simulink model "testemplanner_cs"  (R2023a)
settings: Solver=ode5  StartTime=0.0  StopTime=60  FixedStep=1/1000  RelTol=1e-3
PreLoadFcn:
  | mbxruntime.callbacks.PreLoadFcn(bdroot);
PostLoadFcn:
  | mbxruntime.callbacks.PostLoadFcn(bdroot);
InitFcn:
  | mbxruntime.callbacks.InitFcn(bdroot);
StartFcn:
  | mbxruntime.callbacks.StartFcn(bdroot);
StopFcn:
  | mbxruntime.callbacks.StopFcn(bdroot);
model workspace (MAT data in the model file):
  mbox_table : object (value not decoded)
  model_closed = 0
  sim_status = 0
undefined symbols (not defined in the file): aubr, c_factor, cf, cr, DiscIntNeverNeededParam, global_path_x, global_path_y, KD_PID_distance, KD_PID_speed, KI_PID_distance, KI_PID_speed, KP_PID_distance, KP_PID_speed, la, lb, LQR_K1, LQR_K2, LQR_K3, LQR_K4, m, rack_displacement, right_wheel_ground, tablebr, vubr, vx_break_point
libraries: PreScanSimulinkLibrary x14, Solver_SF x1
(part 4 of 8)

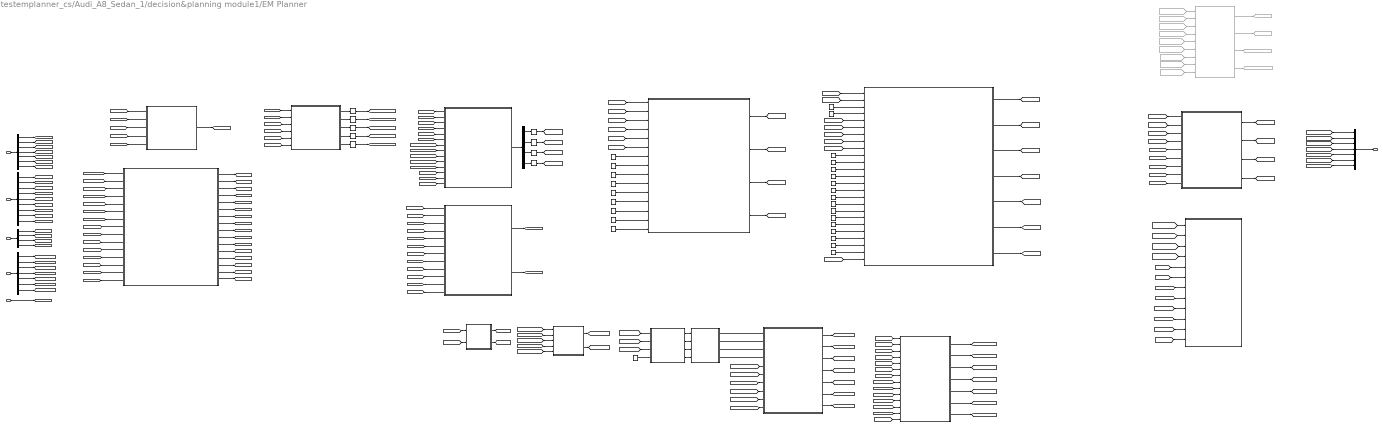
== system testemplanner_cs/Audi_A8_Sedan_1/decision&planning module1/EM Planner ==
  referenceline_info : Inport
  location_info : Inport  Port=2
  perception_info : Inport  Port=3
  pre_planning_info : Inport  Port=4
  current time : Inport  Port=5
  Bus Creator : BusCreator  Inputs=7
  Bus Selector : BusSelector  OutputSignals=referenceline_x,referenceline_y,referenceline_heading,referenceline_kappa,origin_match_point_index,origin_proj_x,origin_proj_y
  Bus Selector1 : BusSelector  OutputSignals=host_x,host_y,host_heading_xy,host_vx,host_vy,host_yawrate,host_speed,host_ax,host_ay
  Bus Selector2 : BusSelector  OutputSignals=obs_x_set_gcs,obs_y_set_gcs,obs_velocity_set_gcs,obs_heading_set_gcs
  Bus Selector3 : BusSelector  OutputSignals=trajectory_x_gcs,trajectory_y_gcs,trajectory_heading_gcs,trajectory_kappa_gcs,trajectory_speed_gcs,trajectory_accel_gcs,trajectory_time_gcs
  Bus Selector4 : BusSelector  OutputSignals=s_set,l_set,dl_set,ddl_set
  Cartesian2Frenet-panning start point : Subsystem
  Constant : Constant  Value=11
  Constant1 : Constant  Value=4
  Constant10 : Constant  Value=5
  Constant11 : Constant  Value=2
  Constant12 : Constant  Value=2
  Constant13 : Constant  Value=25000
  Constant14 : Constant  Value=50
  Constant15 : Constant  Value=20
  Constant16 : Constant  Value=25
  Constant{2,17..19} (4 alike) : Constant  Value=15
  Constant20 : Constant  Value=3
  Constant21 : Constant  Value=3
  Constant22 : Constant  Value=1.63
  Constant23 : Constant  Value=0.1
  Constant24 : Constant  Value=-0.1
  Constant25 : Constant  Value=0.02
  Constant26 : Constant  Value=-0.02
  Constant3 : Constant
  Constant4 : Constant  Value=2000
  Constant5 : Constant  Value=2
  Constant6 : Constant  Value=3
  Constant7 : Constant  Value=10
  Constant8 : Constant  Value=1e6
  Constant9 : Constant  Value=8
  Dynamic Programming&Increase DP Node : Subsystem
  Frenet2Cartesian : MATLAB Function  TreatAsAtomicUnit=on
  Frenet2Cartesian task : MATLAB Function  Commented=on  TreatAsAtomicUnit=on
  From144 : From  Commented=on  GotoTag=qp_path_s
  From151 : From  Commented=on  GotoTag=qp_path_l
  From152 : From  Commented=on  GotoTag=qp_path_dl
  From153 : From  Commented=on  GotoTag=qp_path_ddl
  From154 : From  Commented=on  GotoTag=referenceline_x
  From155 : From  Commented=on  GotoTag=referenceline_y
  From156 : From  Commented=on  GotoTag=referenceline_heading
  From157 : From  Commented=on  GotoTag=referenceline_kappa
  From158 : From  Commented=on  GotoTag=index2s
  Generate Convex Space&Quadratic Programming : Subsystem
  Goto101 : Goto  Commented=on  GotoTag=trajectory_x_init
  Goto102 : Goto  Commented=on  GotoTag=trajectory_y_init
  Goto103 : Goto  Commented=on  GotoTag=trajectory_heading_init
  Goto104 : Goto  Commented=on  GotoTag=trajectory_kappa_init
  Obs : Subsystem
  Selector{1..9} (9 alike) : Selector  InputPortWidth=128  IndexOptions=Index vector (dialog)  Indices=1  OutputSizes=1
  cacul planning start gcs : MATLAB Function  TreatAsAtomicUnit=on
  calc path length and map between point and s : MATLAB Function  TreatAsAtomicUnit=on
  calc speed planning start condition : MATLAB Function  TreatAsAtomicUnit=on
  generate index2s : MATLAB Function  TreatAsAtomicUnit=on
  increase st point count : MATLAB Function  TreatAsAtomicUnit=on
  match&proj point search2 : MATLAB Function  TreatAsAtomicUnit=on
  path and speed merge : MATLAB Function  TreatAsAtomicUnit=on
  plot1 : MATLAB Function  TreatAsAtomicUnit=on
  simple speed qp planning : MATLAB Function  TreatAsAtomicUnit=on
  stitch trajectory : MATLAB Function  TreatAsAtomicUnit=on
  EM Planner result : Outport
  wires:
  referenceline_info/1 -> Bus Selector/1
  Bus Selector/1 -> [referenceline_x]  "<referenceline_x>"
  Bus Selector/2 -> [referenceline_y]  "<referenceline_y>"
  Bus Selector/3 -> [referenceline_heading]  "<referenceline_heading>"
  Bus Selector/4 -> [referenceline_kappa]  "<referenceline_kappa>"
  location_info/1 -> Bus Selector1/1
  Bus Selector1/1 -> [host_x]  "<host_x>"
  Bus Selector1/2 -> [host_y]  "<host_y>"
  Bus Selector1/3 -> [host_heading_xy]  "<host_heading_xy>"
  Bus Selector1/4 -> [host_vx_vcs]  "<host_vx>"
  Bus Selector1/5 -> [host_vy_vcs]  "<host_vy>"
  Bus Selector1/6 -> [host_yawrate]  "<host_yawrate>"
  Bus Selector1/7 -> [host_speed]  "<host_speed>"
  Bus Selector1/8 -> [host_ax_vcs]  "<host_ax>"
  Bus Selector1/9 -> [host_ay_vcs]  "<host_ay>"
  perception_info/1 -> Bus Selector2/1
  Bus Selector2/1 -> [obs_x_set_gcs]  "<obs_x_set_gcs>"
  Bus Selector2/2 -> [obs_y_set_gcs]  "<obs_y_set_gcs>"
  Bus Selector2/3 -> [obs_velocity_set_gcs]  "<obs_velocity_set_gcs>"
  Bus Selector2/4 -> [obs_heading_set_gcs]  "<obs_heading_set_gcs>"
  pre_planning_info/1 -> Bus Selector3/1
  Bus Selector3/1 -> [pre_trajectory_x_gcs]  "<trajectory_x_gcs>"
  Bus Selector3/2 -> [pre_trajectory_y_gcs]  "<trajectory_y_gcs>"
  Bus Selector3/3 -> [pre_trajectory_heading_gcs]  "<trajectory_heading_gcs>"
  Bus Selector3/4 -> [pre_trajectory_kappa_gcs]  "<trajectory_kappa_gcs>"
  Bus Selector3/5 -> [pre_trajectory_speed_gcs]  "<trajectory_speed_gcs>"
  Bus Selector3/6 -> [pre_trajectory_accel_gcs]  "<trajectory_accel_gcs>"
  current time/1 -> [current_time]
  [pre_trajectory_x_gcs] -> cacul planning start gcs/1(pre_trajectory_x)
  [pre_trajectory_y_gcs] -> cacul planning start gcs/2(pre_trajectory_y)
  [pre_trajectory_heading_gcs] -> cacul planning start gcs/3(pre_trajectory_heading)
  [pre_trajectory_kappa_gcs] -> cacul planning start gcs/4(pre_trajectory_kappa)
  [pre_trajectory_speed_gcs] -> cacul planning start gcs/5(pre_trajectory_speed)
  [pre_trajectory_accel_gcs] -> cacul planning start gcs/6(pre_trajectory_accel)
  [pre_trajectory_time] -> cacul planning start gcs/7(pre_trajectory_time)
  [current_time] -> cacul planning start gcs/8(current_time)
  [host_x] -> cacul planning start gcs/9(host_x)
  [host_y] -> cacul planning start gcs/10(host_y)
  [host_heading_xy] -> cacul planning start gcs/11(host_heading_xy)
  [host_vx_vcs] -> cacul planning start gcs/12(host_vx)
  [host_vy_vcs] -> cacul planning start gcs/13(host_vy)
  [host_ax_vcs] -> cacul planning start gcs/14(host_ax)
  [host_ay_vcs] -> cacul planning start gcs/15(host_ay)
  cacul planning start gcs/1(planning_start_x) -> [planning_start_x]
  cacul planning start gcs/2(planning_start_y) -> [planning_start_y]
  cacul planning start gcs/3(planning_start_heading) -> [planning_start_heading]
  cacul planning start gcs/4(planning_start_kappa) -> [planning_start_kappa]
  cacul planning start gcs/5(planning_start_vx) -> [planning_start_vx]
  cacul planning start gcs/6(planning_start_vy) -> [planning_start_vy]
  cacul planning start gcs/7(planning_start_ax) -> [planning_start_ax]
  cacul planning start gcs/8(planning_start_ay) -> [planning_start_ay]
  cacul planning start gcs/9(planning_start_time) -> [planning_start_time]
  cacul planning start gcs/10(stitch_x) -> [stitch_x]
  cacul planning start gcs/11(stitch_y) -> [stitch_y]
  cacul planning start gcs/12(stitch_heading) -> [stitch_heading]
  cacul planning start gcs/13(stitch_kappa) -> [stitch_kappa]
  cacul planning start gcs/14(stitch_speed) -> [stitch_speed]
  cacul planning start gcs/15(stitch_accel) -> [stitch_accel]
  cacul planning start gcs/16(stitch_time) -> [stitch_time]
  Bus Selector/5 -> [origin_match_point_index]  "<origin_match_point_index>"
  Bus Selector/6 -> [origin_proj_x]  "<origin_proj_x>"
  Bus Selector/7 -> [origin_proj_y]  "<origin_proj_y>"
  [origin_match_point_index] -> generate index2s/1(origin_match_point_index)
  [origin_proj_x] -> generate index2s/2(origin_proj_x)
  [origin_proj_y] -> generate index2s/3(origin_proj_y)
  [referenceline_x] -> generate index2s/4(path_x)
  [referenceline_y] -> generate index2s/5(path_y)
  generate index2s/1(index2s) -> [index2s]
  match&proj point search2/3(proj_y_set) -> Selector3/1
  match&proj point search2/1(match_point_index_set) -> Selector1/1
  match&proj point search2/2(proj_x_set) -> Selector2/1
  match&proj point search2/4(proj_heading_set) -> Selector4/1
  match&proj point search2/5(proj_kappa_set) -> Selector5/1
  [planning_start_x] -> match&proj point search2/1(x_set)
  [planning_start_y] -> match&proj point search2/2(y_set)
  [referenceline_x] -> match&proj point search2/3(frenet_x_set)
  [referenceline_y] -> match&proj point search2/4(frenet_y_set)
  [referenceline_heading] -> match&proj point search2/5(frenet_heading_set)
  [referenceline_kappa] -> match&proj point search2/6(frenet_kapppa_set)
  Selector1/1 -> [planning_start_match_point_index]
  Selector2/1 -> [planning_start_proj_x]
  Selector3/1 -> [planning_start_proj_y]
  Selector4/1 -> [planning_start_proj_heading]
  Selector5/1 -> [planning_start_proj_kappa]
  Cartesian2Frenet-panning start point/1(Caetesian2Frenetout) -> Bus Selector4/1
  Bus Selector4/1 -> Selector6/1  "<s_set>"
  Bus Selector4/2 -> Selector7/1  "<l_set>"
  Bus Selector4/3 -> Selector8/1  "<dl_set>"
  Bus Selector4/4 -> Selector9/1  "<ddl_set>"
  [planning_start_x] -> Cartesian2Frenet-panning start point/1(x_set)
  [planning_start_y] -> Cartesian2Frenet-panning start point/2(y_set)
  [planning_start_vx] -> Cartesian2Frenet-panning start point/3(vx_set)
  [planning_start_vy] -> Cartesian2Frenet-panning start point/4(vy_set)
  [planning_start_ax] -> Cartesian2Frenet-panning start point/5(ax_set)
  [planning_start_ay] -> Cartesian2Frenet-panning start point/6(ay_set)
  [planning_start_proj_x] -> Cartesian2Frenet-panning start point/7(proj_x_set)
  [planning_start_proj_y] -> Cartesian2Frenet-panning start point/8(proj_y_set)
  [planning_start_proj_heading] -> Cartesian2Frenet-panning start point/9(proj_heading_set)
  [planning_start_proj_kappa] -> Cartesian2Frenet-panning start point/10(proj_kappa_set)
  [planning_start_match_point_index] -> Cartesian2Frenet-panning start point/11(match_point_index_set)
  [referenceline_x] -> Cartesian2Frenet-panning start point/12(frenet_x_set)
  [referenceline_y] -> Cartesian2Frenet-panning start point/13(frenet_y_set)
  [index2s] -> Cartesian2Frenet-panning start point/14(index2s)
  Selector6/1 -> [planning_start_s]
  Selector7/1 -> [planning_start_l]
  Selector8/1 -> [planning_start_dl]
  Selector9/1 -> [planning_start_ddl]
  [host_x] -> Obs/1(host_x)
  [host_y] -> Obs/2(host_y)
  [obs_x_set_gcs] -> Obs/3(obs_x_set_gcs)
  [obs_y_set_gcs] -> Obs/4(obs_y_set_gcs)
  [obs_velocity_set_gcs] -> Obs/5(obs_velocity_set_gcs)
  [obs_heading_set_gcs] -> Obs/6(obs_heading_set_gcs)
  [host_heading_xy] -> Obs/7(host_heading_xy)
  [index2s] -> Obs/12(index2s)
  [referenceline_x] -> Obs/8(referenceline_x)
  [referenceline_y] -> Obs/9(referenceline_y)
  [referenceline_heading] -> Obs/10(referenceline_heading)
  [referenceline_kappa] -> Obs/11(referenceline_kappa)
  Obs/1(static_obs_s_set) -> [static_obs_s_set]
  Obs/2(static_obs_l_set) -> [static_obs_l_set]
  [qp_path_s] -> Frenet2Cartesian/1(s_set)
  [qp_path_l] -> Frenet2Cartesian/2(l_set)
  [qp_path_dl] -> Frenet2Cartesian/3(dl_set)
  [qp_path_ddl] -> Frenet2Cartesian/4(ddl_set)
  [referenceline_x] -> Frenet2Cartesian/5(frenet_x)
  [referenceline_y] -> Frenet2Cartesian/6(frenet_y)
  [referenceline_heading] -> Frenet2Cartesian/7(frenet_heading)
  [index2s] -> Frenet2Cartesian/9(index2s)
  [referenceline_kappa] -> Frenet2Cartesian/8(frenet_kappa)
  Frenet2Cartesian/1(x_point_set) -> [trajectory_x_init]
  Frenet2Cartesian/2(y_point_set) -> [trajectory_y_init]
  Frenet2Cartesian/3(heading_point_set) -> [trajectory_heading_init]
  Frenet2Cartesian/4(kappa_point_set) -> [trajectory_kappa_init]
  stitch trajectory/6(trajectory_accel_final) -> [trajectory_accel_final]
  stitch trajectory/7(trajectory_time_final) -> [trajectory_time_final]
  [trajectory_heading] -> stitch trajectory/3(trajectory_heading)
  [planning_start_time] -> path and speed merge/5(current_time)
  increase st point count/2(s_dot) -> path and speed merge/2(s_dot)
  [plan_start_s_dot] -> simple speed qp planning/1(plan_start_s_dot)
  [trajectory_x_final] -> Bus Creator/1  "trajectory_x_gcs"
  [stitch_kappa] -> stitch trajectory/11(stitch_kappa)
  [trajectory_y_final] -> Bus Creator/2  "trajectory_y_gcs"
  simple speed qp planning/4(relative_time_init) -> increase st point count/4(relative_time_init)
  path and speed merge/5(trajectory_speed) -> [trajectory_speed]
  simple speed qp planning/3(s_dot2_init) -> increase st point count/3(s_dot2_init)
  increase st point count/4(relative_time) -> path and speed merge/4(relative_time)
  [plan_start_s_dot2] -> simple speed qp planning/2(plan_start_s_dot2)
  simple speed qp planning/1(s_init) -> increase st point count/1(s_init)
  [trajectory_heading_init] -> path and speed merge/9(trajectory_heading_init)
  path and speed merge/7(trajectory_time) -> [trajectory_time]
  [trajectory_x] -> stitch trajectory/1(trajectory_x)
  path and speed merge/6(trajectory_accel) -> [trajectory_accel]
  [stitch_speed] -> stitch trajectory/12(stitch_speed)
  [trajectory_y] -> stitch trajectory/2(trajectory_y)
  [stitch_accel] -> stitch trajectory/13(stitch_accel)
  stitch trajectory/3(trajectory_heading_final) -> [trajectory_heading_final]
  [trajectory_x_init] -> path and speed merge/7(trajectory_x_init)
  [path_s] -> path and speed merge/6(path_s)
  [path_s_end] -> simple speed qp planning/3(s_end)
  calc speed planning start condition/2(plan_start_s_dot2) -> [plan_start_s_dot2]
  stitch trajectory/5(trajectory_speed_final) -> [trajectory_speed_final]
  Constant9/1 -> simple speed qp planning/4(recommend_T)
  [trajectory_time] -> stitch trajectory/7(trajectory_time)
  [stitch_time] -> stitch trajectory/14(stitch_time)
  [planning_start_ay] -> calc speed planning start condition/4(plan_start_ay)
  [trajectory_accel] -> stitch trajectory/6(trajectory_accel)
  [stitch_heading] -> stitch trajectory/10(stitch_heading)
  [trajectory_kappa] -> stitch trajectory/4(trajectory_kappa)
  [trajectory_heading_final] -> Bus Creator/3  "trajectory_heading_gcs"
  [trajectory_speed_final] -> Bus Creator/5  "trajectory_speed_gcs"
  increase st point count/3(s_dot2) -> path and speed merge/3(s_dot2)
  calc path length and map between point and s/2(path_s) -> [path_s]
  [trajectory_time_final] -> Bus Creator/7  "trajectory_time_gcs"
  stitch trajectory/4(trajectory_kappa_final) -> [trajectory_kappa_final]
  calc path length and map between point and s/1(path_s_end) -> [path_s_end]
  [planning_start_vy] -> calc speed planning start condition/2(plan_start_vy)
  increase st point count/1(s) -> path and speed merge/1(s)
  [planning_start_heading] -> calc speed planning start condition/5(plan_start_heading)
  [trajectory_accel_final] -> Bus Creator/6  "trajectory_accel_gcs"
  path and speed merge/4(trajectory_kappa) -> [trajectory_kappa]
  [stitch_y] -> stitch trajectory/9(stitch_y)
  path and speed merge/1(trajectory_x) -> [trajectory_x]
  stitch trajectory/1(trajectory_x_final) -> [trajectory_x_final]
  [trajectory_x_init] -> calc path length and map between point and s/1(trajectory_x)
  stitch trajectory/2(trajectory_y_final) -> [trajectory_y_final]
  calc speed planning start condition/1(plan_start_s_dot) -> [plan_start_s_dot]
  [trajectory_y_init] -> calc path length and map between point and s/2(trajectory_y)
  [trajectory_speed] -> stitch trajectory/5(trajectory_speed)
  [trajectory_kappa_init] -> path and speed merge/10(trajectory_kappa_init)
  [planning_start_vx] -> calc speed planning start condition/1(plan_start_vx)
  [trajectory_y_init] -> path and speed merge/8(trajectory_y_init)
  path and speed merge/2(trajectory_y) -> [trajectory_y]
  path and speed merge/3(trajectory_heading) -> [trajectory_heading]
  Bus Creator/1 -> EM Planner result/1
  [stitch_x] -> stitch trajectory/8(stitch_x)
  simple speed qp planning/2(s_dot_init) -> increase st point count/2(s_dot_init)
  [planning_start_ax] -> calc speed planning start condition/3(plan_start_ax)
  [trajectory_kappa_final] -> Bus Creator/4  "trajectory_kappa_gcs"
  Bus Selector3/7 -> [pre_trajectory_time]  "<trajectory_time_gcs>"
  From158/1 -> Frenet2Cartesian task/9(index2s)
  From156/1 -> Frenet2Cartesian task/7(frenet_path_heading)
  Frenet2Cartesian task/1(x_set) -> Goto101/1
  Frenet2Cartesian task/4(kappa_set) -> Goto104/1
  From157/1 -> Frenet2Cartesian task/8(frenet_path_kappa)
  Frenet2Cartesian task/2(y_set) -> Goto102/1
  From144/1 -> Frenet2Cartesian task/1(s_set)
  From154/1 -> Frenet2Cartesian task/5(frenet_path_x)
  From152/1 -> Frenet2Cartesian task/3(dl_set)
  From151/1 -> Frenet2Cartesian task/2(l_set)
  From155/1 -> Frenet2Cartesian task/6(frenet_path_y)
  From153/1 -> Frenet2Cartesian task/4(ddl_set)
  Frenet2Cartesian task/3(heading_set) -> Goto103/1
  [static_obs_s_set] -> plot1/7(obs_s_set)
  [planning_start_s] -> plot1/9(start_s)
  [l_min] -> plot1/5(l_min)
  [dp_path_l_final] -> plot1/2(dp_l)
  [planning_start_dl] -> plot1/11(start_dl)
  [dp_path_s_final] -> plot1/1(dp_s)
  [planning_start_l] -> plot1/10(start_l)
  [static_obs_l_set] -> plot1/8(obs_l_set)
  [qp_path_s] -> plot1/3(qp_s)
  [qp_path_l] -> plot1/4(qp_l)
  [l_max] -> plot1/6(l_max)
  [planning_start_s] -> Dynamic Programming&Increase DP Node/1(plan_start_s)
  [planning_start_l] -> Dynamic Programming&Increase DP Node/2(plan_start_l)
  [planning_start_dl] -> Dynamic Programming&Increase DP Node/3(plan_start_dl)
  [planning_start_ddl] -> Dynamic Programming&Increase DP Node/4(plan_start_ddl)
  [static_obs_s_set] -> Dynamic Programming&Increase DP Node/5(static_obs_s_set)
  [static_obs_l_set] -> Dynamic Programming&Increase DP Node/6(static_obs_l_set)
  Constant/1 -> Dynamic Programming&Increase DP Node/7(row)
  Constant1/1 -> Dynamic Programming&Increase DP Node/8(col)
  Constant2/1 -> Dynamic Programming&Increase DP Node/9(sample_s)
  Constant3/1 -> Dynamic Programming&Increase DP Node/10(sample_l)
  Constant4/1 -> Dynamic Programming&Increase DP Node/11(dp_dl_cost)
  Constant5/1 -> Dynamic Programming&Increase DP Node/12(dp_ddl_cost)
  Constant6/1 -> Dynamic Programming&Increase DP Node/13(dp_dddl_cost)
  Constant7/1 -> Dynamic Programming&Increase DP Node/14(dp_l_cost)
  Constant8/1 -> Dynamic Programming&Increase DP Node/15(dp_obs_cost)
  Dynamic Programming&Increase DP Node/1(dp_path_s_final) -> [dp_path_s_final]
  Dynamic Programming&Increase DP Node/2(dp_path_l_final) -> [dp_path_l_final]
  Dynamic Programming&Increase DP Node/3(dp_path_dl_final) -> [dp_path_dl_final]
  Dynamic Programming&Increase DP Node/4(dp_path_ddl_final) -> [dp_path_ddl_final]
  [static_obs_l_set] -> Generate Convex Space&Quadratic Programming/2(static_obs_l_set)
  [static_obs_s_set] -> Generate Convex Space&Quadratic Programming/1(static_obs_s_set)
  Constant10/1 -> Generate Convex Space&Quadratic Programming/3(static_obs_length)
  Constant11/1 -> Generate Convex Space&Quadratic Programming/4(static_obs_width)
  [dp_path_s_final] -> Generate Convex Space&Quadratic Programming/5(dp_path_s_final)
  [dp_path_l_final] -> Generate Convex Space&Quadratic Programming/6(dp_path_l_final)
  [planning_start_l] -> Generate Convex Space&Quadratic Programming/7(plan_start_l)
  [planning_start_dl] -> Generate Convex Space&Quadratic Programming/8(plan_start_dl)
  [planning_start_ddl] -> Generate Convex Space&Quadratic Programming/9(plan_start_ddl)
  Constant12/1 -> Generate Convex Space&Quadratic Programming/10(qp_l_cost)
  Constant13/1 -> Generate Convex Space&Quadratic Programming/11(qp_dl_cost)
  Constant14/1 -> Generate Convex Space&Quadratic Programming/12(qp_ddl_cost)
  Constant15/1 -> Generate Convex Space&Quadratic Programming/13(qp_dddl_cost)
  Constant16/1 -> Generate Convex Space&Quadratic Programming/14(qp_centre_cost)
  Constant17/1 -> Generate Convex Space&Quadratic Programming/15(qp_end_l_cost)
  Constant18/1 -> Generate Convex Space&Quadratic Programming/16(qp_end_dl_cost)
  Constant19/1 -> Generate Convex Space&Quadratic Programming/17(qp_end_ddl_cost)
  Constant20/1 -> Generate Convex Space&Quadratic Programming/18(host_d1)
  Constant21/1 -> Generate Convex Space&Quadratic Programming/19(host_d2)
  Constant22/1 -> Generate Convex Space&Quadratic Programming/20(host_width)
  Generate Convex Space&Quadratic Programming/1(qp_path_l) -> [qp_path_l]
  Generate Convex Space&Quadratic Programming/2(qp_path_dl) -> [qp_path_dl]
  Generate Convex Space&Quadratic Programming/3(qp_path_ddl) -> [qp_path_ddl]
  Generate Convex Space&Quadratic Programming/4(l_min) -> [l_min]
  Generate Convex Space&Quadratic Programming/5(l_max) -> [l_max]
  Generate Convex Space&Quadratic Programming/6(qp_path_s) -> [qp_path_s]
  [planning_start_s] -> Generate Convex Space&Quadratic Programming/25(plan_start_s)
  Constant23/1 -> Generate Convex Space&Quadratic Programming/21(delta_dl_max)
  Constant24/1 -> Generate Convex Space&Quadratic Programming/22(delta_dl_min)
  Constant25/1 -> Generate Convex Space&Quadratic Programming/23(delta_ddl_max)
  Constant26/1 -> Generate Convex Space&Quadratic Programming/24(delta_ddl_min)
  Generate Convex Space&Quadratic Programming/7(centre_line) -> [centre_line]
  [centre_line] -> plot1/12(centre_line)

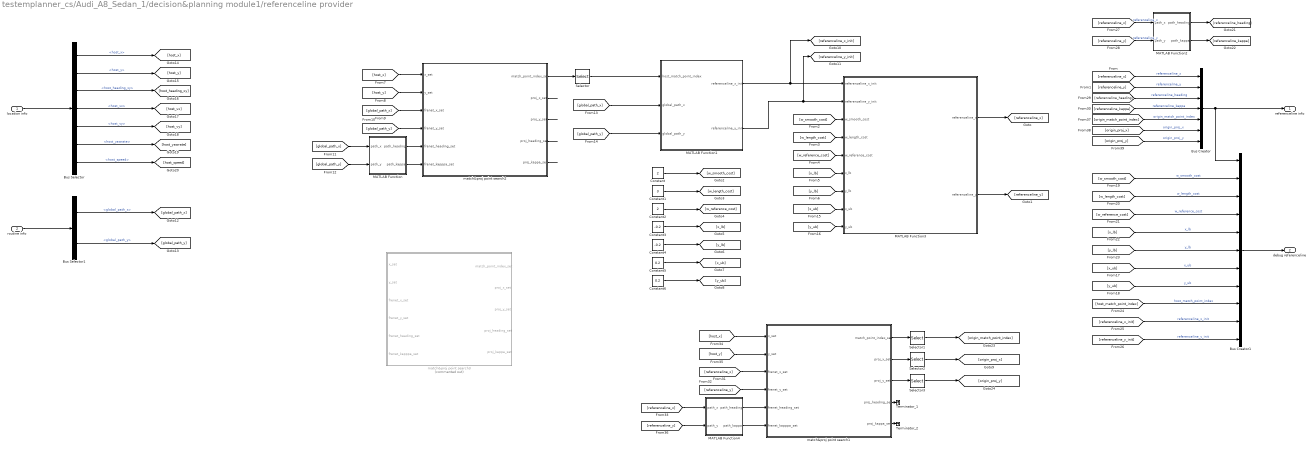
== system testemplanner_cs/Audi_A8_Sedan_1/decision&planning module1/referenceline provider ==
  location info : Inport
  routine info : Inport  Port=2
  Bus Creator : BusCreator  Inputs=7
  Bus Creator1 : BusCreator  Inputs=11
  Bus Selector : BusSelector  OutputSignals=host_x,host_y,host_heading_xy,host_vx,host_vy,host_yawrate,host_speed
  Bus Selector1 : BusSelector  OutputSignals=global_path_x,global_path_y
  Constant : Constant  Value=2
  Constant1 : Constant  Value=3
  Constant2 : Constant  Value=2
  Constant3 : Constant  Value=-0.2
  Constant4 : Constant  Value=-0.2
  Constant5 : Constant  Value=0.2
  Constant6 : Constant  Value=0.2
  MATLAB Function : MATLAB Function  TreatAsAtomicUnit=on
  MATLAB Function1 : MATLAB Function  TreatAsAtomicUnit=on
  MATLAB Function2 : MATLAB Function  TreatAsAtomicUnit=on
  MATLAB Function3 : MATLAB Function  TreatAsAtomicUnit=on
  MATLAB Function4 : MATLAB Function  TreatAsAtomicUnit=on
  Selector{,1..3} (4 alike) : Selector  InputPortWidth=128  IndexOptions=Index vector (dialog)  Indices=1  OutputSizes=1
  Terminator_1 : Terminator
  Terminator_2 : Terminator
  match&proj point search1 : MATLAB Function  TreatAsAtomicUnit=on
  match&proj point search2 : MATLAB Function  TreatAsAtomicUnit=on
  match&proj point search3 : MATLAB Function  Commented=on  TreatAsAtomicUnit=on
  referenceline info : Outport
  debug referenceline : Outport  Port=2
  wires:
  [x_lb] -> MATLAB Function3/6(x_lb)
  [global_path_x] -> MATLAB Function/1(path_x)
  [global_path_x] -> match&proj point search2/3(frenet_x_set)
  [w_reference_cost] -> MATLAB Function3/5(w_reference_cost)
  MATLAB Function1/1(referenceline_x_init) -> [referenceline_x_init], MATLAB Function3/1(referenceline_x_init)
  [w_smooth_cost] -> MATLAB Function3/3(w_smooth_cost)
  [host_y] -> match&proj point search2/2(y_set)
  match&proj point search2/1(match_point_index_set) -> Selector/1
  [global_path_y] -> MATLAB Function/2(path_y)
  MATLAB Function/2(path_kappa) -> match&proj point search2/6(frenet_kapppa_set)
  Constant4/1 -> [y_lb]
  [global_path_x] -> MATLAB Function1/2(global_path_x)
  MATLAB Function/1(path_heading) -> match&proj point search2/5(frenet_heading_set)
  [global_path_y] -> MATLAB Function1/3(global_path_y)
  Selector/1 -> MATLAB Function1/1(host_match_point_index)
  Constant2/1 -> [w_reference_cost]
  [global_path_y] -> match&proj point search2/4(frenet_y_set)
  [host_x] -> match&proj point search2/1(x_set)
  [w_length_cost] -> MATLAB Function3/4(w_length_cost)
  MATLAB Function1/2(referenceline_y_init) -> [referenceline_y_init], MATLAB Function3/2(referenceline_y_init)
  Constant/1 -> [w_smooth_cost]
  Constant1/1 -> [w_length_cost]
  Constant3/1 -> [x_lb]
  [x_ub] -> MATLAB Function3/8(x_ub)
  [y_lb] -> MATLAB Function3/7(y_lb)
  [y_ub] -> MATLAB Function3/9(y_ub)
  Constant6/1 -> [y_ub]
  Constant5/1 -> [x_ub]
  MATLAB Function3/1(referenceline_x) -> [referenceline_x]
  MATLAB Function3/2(referenceline_y) -> [referenceline_y]
  Bus Creator/1 -> Bus Creator1/1, referenceline info/1
  [referenceline_y] -> Bus Creator/2  "referenceline_y"
  [referenceline_x] -> Bus Creator/1  "referenceline_x"
  Bus Creator1/1 -> debug referenceline/1
  [w_smooth_cost] -> Bus Creator1/2  "w_smooth_cost"
  [w_length_cost] -> Bus Creator1/3  "w_length_cost"
  [w_reference_cost] -> Bus Creator1/4  "w_reference_cost"
  [x_lb] -> Bus Creator1/5  "x_lb"
  [y_lb] -> Bus Creator1/6  "y_lb"
  [x_ub] -> Bus Creator1/7  "x_ub"
  [y_ub] -> Bus Creator1/8  "y_ub"
  [host_match_point_index] -> Bus Creator1/9  "host_match_point_index"
  [referenceline_x_init] -> Bus Creator1/10  "referenceline_x_init"
  [referenceline_y_init] -> Bus Creator1/11  "referenceline_y_init"
  Bus Selector1/2 -> [global_path_y]  "<global_path_y>"
  Bus Selector1/1 -> [global_path_x]  "<global_path_x>"
  routine info/1 -> Bus Selector1/1
  Bus Selector/7 -> [host_speed]  "<host_speed>"
  Bus Selector/6 -> [host_yawrate]  "<host_yawrate>"
  Bus Selector/2 -> [host_y]  "<host_y>"
  Bus Selector/1 -> [host_x]  "<host_x>"
  Bus Selector/3 -> [host_heading_xy]  "<host_heading_xy>"
  Bus Selector/4 -> [host_vx]  "<host_vx>"
  Bus Selector/5 -> [host_vy]  "<host_vy>"
  location info/1 -> Bus Selector/1
  [referenceline_y] -> MATLAB Function2/2(path_y)  "referenceline_y"
  [referenceline_x] -> MATLAB Function2/1(path_x)  "referenceline_x"
  MATLAB Function2/1(path_heading) -> [referenceline_heading]
  MATLAB Function2/2(path_kappa) -> [referenceline_kappa]
  [referenceline_heading] -> Bus Creator/3  "referenceline_heading"
  [referenceline_kappa] -> Bus Creator/4  "referenceline_kappa"
  [host_x] -> match&proj point search1/1(x_set)
  [referenceline_y] -> match&proj point search1/4(frenet_y_set)
  MATLAB Function4/1(path_heading) -> match&proj point search1/5(frenet_heading_set)
  MATLAB Function4/2(path_kappa) -> match&proj point search1/6(frenet_kapppa_set)
  [referenceline_y] -> MATLAB Function4/2(path_y)
  [host_y] -> match&proj point search1/2(y_set)
  [referenceline_x] -> match&proj point search1/3(frenet_x_set)
  [referenceline_x] -> MATLAB Function4/1(path_x)
  match&proj point search1/1(match_point_index_set) -> Selector1/1
  Selector1/1 -> [origin_match_point_index]
  match&proj point search1/2(proj_x_set) -> Selector2/1
  Selector2/1 -> [origin_proj_x]
  match&proj point search1/3(proj_y_set) -> Selector3/1
  Selector3/1 -> [origin_proj_y]
  [origin_match_point_index] -> Bus Creator/5  "origin_match_point_index"
  [origin_proj_x] -> Bus Creator/6  "origin_proj_x"
  [origin_proj_y] -> Bus Creator/7  "origin_proj_y"
  match&proj point search2/2(proj_x_set) -> ?
  match&proj point search2/3(proj_y_set) -> ?
  match&proj point search2/4(proj_heading_set) -> ?
  match&proj point search2/5(proj_kappa_set) -> ?
  match&proj point search1/4(proj_heading_set) -> Terminator_1/1
  match&proj point search1/5(proj_kappa_set) -> Terminator_2/1

== system testemplanner_cs/Box_1/Dynamics_Empty/MuxState ==
  note: mode: Dynamics
  note: mode: Positioning
  note: mode: Dynamics
      | VelVEHICLE
      | wrt VEH
  note: AnglesVEHICLE
      | wrtGLOB
  note: For state mode 'Dynamic' positions
      | are not taken into account, as they
      | are computed by integrating velocity.
      | Click annotation for Help.
  x [m] : Inport  SampleTime=TimeStep
  y [m] : Inport  Port=2  SampleTime=TimeStep
  z [m] : Inport  Port=3  SampleTime=TimeStep
  dx [m/s] : Inport  Port=4  SampleTime=TimeStep
  dy [m/s] : Inport  Port=5  SampleTime=TimeStep
  dz [m/s] : Inport  Port=6  SampleTime=TimeStep
  R [rad] : Inport  Port=7  SampleTime=TimeStep
  P [rad] : Inport  Port=8  SampleTime=TimeStep
  Y [rad] : Inport  Port=9  SampleTime=TimeStep
  Constant : Constant  DisableCoverage=on  Value=positioningmode
  Discrete-Time Integrator : DiscreteIntegrator  SampleTime=TimeStep  ICPrevOutput=DiscIntNeverNeededParam  ICPrevScaledInput=DiscIntNeverNeededParam
  Ground : Ground
  Ground1 : Ground
  Mux1 : Mux  Inputs=[3 3]
  Mux2 : Mux  Inputs=3
  Mux3 : Mux  Inputs=3
  Mux4 : Mux  Inputs=3
  Mux5 : Mux  Inputs=[3 3]
  Mux6 : Mux  Inputs=[6 3]
  Switch : Switch  Threshold=0.5  SaturateOnIntegerOverflow=off  InputSameDT=off
  Transformation_BODY2GLOBAL : PreScanSimulinkLibrary/Simple_Vehicle_Dynamics/Chassis/MuxDynState/Transformation_BODY2GLOBAL  SystemSampleTime=-1  VariantActivationTime=update diagram  Latency=0  AutoFrameSizeCalculation=off
  mux3 : Mux  Inputs=3
  state : Outport
  wires:
  Constant/1 -> Switch/2
  Mux6/1 -> state/1
  Mux4/1 -> Mux1/1
  Mux5/1 -> Switch/3
  Mux1/1 -> Switch/1
  Switch/1 -> Mux6/1  "PosVeh wrt  GLOB"
  P [rad]/1 -> Mux3/2
  R [rad]/1 -> Mux3/1
  dz [m/s]/1 -> Mux2/3
  dy [m/s]/1 -> Mux2/2
  dx [m/s]/1 -> Mux2/1
  z [m]/1 -> Mux4/3
  y [m]/1 -> Mux4/2
  x [m]/1 -> Mux4/1
  Ground1/1 -> mux3/2  "pitch"
  Y [rad]/1 -> mux3/3, Mux3/3  "yaw"
  Mux3/1 -> Mux6/2
  Transformation_BODY2GLOBAL/1 -> Discrete-Time Integrator/1, Mux5/2  "VelVEH wrt  GLOB"
  mux3/1 -> Transformation_BODY2GLOBAL/2
  Ground/1 -> mux3/1  "roll"
  Mux2/1 -> Mux1/2, Transformation_BODY2GLOBAL/1
  Discrete-Time Integrator/1 -> Mux5/1  "PosVEH wrt  GLOB"

== system testemplanner_cs/Box_1/SELF_Demux/compas converter ==
  rotz [rad] : Inport
  cart2compas : Subsystem
  rad2deg : Gain  Gain=180/pi
  heading [deg] : Outport
  wires:
  rad2deg/1 -> cart2compas/1(Angle [deg])
  rotz [rad]/1 -> rad2deg/1
  cart2compas/1(heading [deg]) -> heading [deg]/1

== system testemplanner_cs/Box_2/Dynamics_Empty/MuxState ==
  note: mode: Dynamics
  note: mode: Positioning
  note: mode: Dynamics
      | VelVEHICLE
      | wrt VEH
  note: AnglesVEHICLE
      | wrtGLOB
  note: For state mode 'Dynamic' positions
      | are not taken into account, as they
      | are computed by integrating velocity.
      | Click annotation for Help.
  x [m] : Inport  SampleTime=TimeStep
  y [m] : Inport  Port=2  SampleTime=TimeStep
  z [m] : Inport  Port=3  SampleTime=TimeStep
  dx [m/s] : Inport  Port=4  SampleTime=TimeStep
  dy [m/s] : Inport  Port=5  SampleTime=TimeStep
  dz [m/s] : Inport  Port=6  SampleTime=TimeStep
  R [rad] : Inport  Port=7  SampleTime=TimeStep
  P [rad] : Inport  Port=8  SampleTime=TimeStep
  Y [rad] : Inport  Port=9  SampleTime=TimeStep
  Constant : Constant  DisableCoverage=on  Value=positioningmode
  Discrete-Time Integrator : DiscreteIntegrator  SampleTime=TimeStep  ICPrevOutput=DiscIntNeverNeededParam  ICPrevScaledInput=DiscIntNeverNeededParam
  Ground : Ground
  Ground1 : Ground
  Mux1 : Mux  Inputs=[3 3]
  Mux2 : Mux  Inputs=3
  Mux3 : Mux  Inputs=3
  Mux4 : Mux  Inputs=3
  Mux5 : Mux  Inputs=[3 3]
  Mux6 : Mux  Inputs=[6 3]
  Switch : Switch  Threshold=0.5  SaturateOnIntegerOverflow=off  InputSameDT=off
  Transformation_BODY2GLOBAL : PreScanSimulinkLibrary/Simple_Vehicle_Dynamics/Chassis/MuxDynState/Transformation_BODY2GLOBAL  SystemSampleTime=-1  VariantActivationTime=update diagram  Latency=0  AutoFrameSizeCalculation=off
  mux3 : Mux  Inputs=3
  state : Outport
  wires:
  Constant/1 -> Switch/2
  Mux6/1 -> state/1
  Mux4/1 -> Mux1/1
  Mux5/1 -> Switch/3
  Mux1/1 -> Switch/1
  Switch/1 -> Mux6/1  "PosVeh wrt  GLOB"
  P [rad]/1 -> Mux3/2
  R [rad]/1 -> Mux3/1
  dz [m/s]/1 -> Mux2/3
  dy [m/s]/1 -> Mux2/2
  dx [m/s]/1 -> Mux2/1
  z [m]/1 -> Mux4/3
  y [m]/1 -> Mux4/2
  x [m]/1 -> Mux4/1
  Ground1/1 -> mux3/2  "pitch"
  Y [rad]/1 -> mux3/3, Mux3/3  "yaw"
  Mux3/1 -> Mux6/2
  Transformation_BODY2GLOBAL/1 -> Discrete-Time Integrator/1, Mux5/2  "VelVEH wrt  GLOB"
  mux3/1 -> Transformation_BODY2GLOBAL/2
  Ground/1 -> mux3/1  "roll"
  Mux2/1 -> Mux1/2, Transformation_BODY2GLOBAL/1
  Discrete-Time Integrator/1 -> Mux5/1  "PosVEH wrt  GLOB"

== system testemplanner_cs/Box_2/SELF_Demux/compas converter ==
  rotz [rad] : Inport
  cart2compas : Subsystem
  rad2deg : Gain  Gain=180/pi
  heading [deg] : Outport
  wires:
  rad2deg/1 -> cart2compas/1(Angle [deg])
  rotz [rad]/1 -> rad2deg/1
  cart2compas/1(heading [deg]) -> heading [deg]/1

== system testemplanner_cs/Box_3/Dynamics_Empty/MuxState ==
  note: mode: Dynamics
  note: mode: Positioning
  note: mode: Dynamics
      | VelVEHICLE
      | wrt VEH
  note: AnglesVEHICLE
      | wrtGLOB
  note: For state mode 'Dynamic' positions
      | are not taken into account, as they
      | are computed by integrating velocity.
      | Click annotation for Help.
  x [m] : Inport  SampleTime=TimeStep
  y [m] : Inport  Port=2  SampleTime=TimeStep
  z [m] : Inport  Port=3  SampleTime=TimeStep
  dx [m/s] : Inport  Port=4  SampleTime=TimeStep
  dy [m/s] : Inport  Port=5  SampleTime=TimeStep
  dz [m/s] : Inport  Port=6  SampleTime=TimeStep
  R [rad] : Inport  Port=7  SampleTime=TimeStep
  P [rad] : Inport  Port=8  SampleTime=TimeStep
  Y [rad] : Inport  Port=9  SampleTime=TimeStep
  Constant : Constant  DisableCoverage=on  Value=positioningmode
  Discrete-Time Integrator : DiscreteIntegrator  SampleTime=TimeStep  ICPrevOutput=DiscIntNeverNeededParam  ICPrevScaledInput=DiscIntNeverNeededParam
  Ground : Ground
  Ground1 : Ground
  Mux1 : Mux  Inputs=[3 3]
  Mux2 : Mux  Inputs=3
  Mux3 : Mux  Inputs=3
  Mux4 : Mux  Inputs=3
  Mux5 : Mux  Inputs=[3 3]
  Mux6 : Mux  Inputs=[6 3]
  Switch : Switch  Threshold=0.5  SaturateOnIntegerOverflow=off  InputSameDT=off
  Transformation_BODY2GLOBAL : PreScanSimulinkLibrary/Simple_Vehicle_Dynamics/Chassis/MuxDynState/Transformation_BODY2GLOBAL  SystemSampleTime=-1  VariantActivationTime=update diagram  Latency=0  AutoFrameSizeCalculation=off
  mux3 : Mux  Inputs=3
  state : Outport
  wires:
  Constant/1 -> Switch/2
  Mux6/1 -> state/1
  Mux4/1 -> Mux1/1
  Mux5/1 -> Switch/3
  Mux1/1 -> Switch/1
  Switch/1 -> Mux6/1  "PosVeh wrt  GLOB"
  P [rad]/1 -> Mux3/2
  R [rad]/1 -> Mux3/1
  dz [m/s]/1 -> Mux2/3
  dy [m/s]/1 -> Mux2/2
  dx [m/s]/1 -> Mux2/1
  z [m]/1 -> Mux4/3
  y [m]/1 -> Mux4/2
  x [m]/1 -> Mux4/1
  Ground1/1 -> mux3/2  "pitch"
  Y [rad]/1 -> mux3/3, Mux3/3  "yaw"
  Mux3/1 -> Mux6/2
  Transformation_BODY2GLOBAL/1 -> Discrete-Time Integrator/1, Mux5/2  "VelVEH wrt  GLOB"
  mux3/1 -> Transformation_BODY2GLOBAL/2
  Ground/1 -> mux3/1  "roll"
  Mux2/1 -> Mux1/2, Transformation_BODY2GLOBAL/1
  Discrete-Time Integrator/1 -> Mux5/1  "PosVEH wrt  GLOB"

== system testemplanner_cs/Box_3/SELF_Demux/compas converter ==
  rotz [rad] : Inport
  cart2compas : Subsystem
  rad2deg : Gain  Gain=180/pi
  heading [deg] : Outport
  wires:
  rad2deg/1 -> cart2compas/1(Angle [deg])
  rotz [rad]/1 -> rad2deg/1
  cart2compas/1(heading [deg]) -> heading [deg]/1

== system testemplanner_cs/Box_4/Dynamics_Empty/MuxState ==
  note: mode: Dynamics
  note: mode: Positioning
  note: mode: Dynamics
      | VelVEHICLE
      | wrt VEH
  note: AnglesVEHICLE
      | wrtGLOB
  note: For state mode 'Dynamic' positions
      | are not taken into account, as they
      | are computed by integrating velocity.
      | Click annotation for Help.
  x [m] : Inport  SampleTime=TimeStep
  y [m] : Inport  Port=2  SampleTime=TimeStep
  z [m] : Inport  Port=3  SampleTime=TimeStep
  dx [m/s] : Inport  Port=4  SampleTime=TimeStep
  dy [m/s] : Inport  Port=5  SampleTime=TimeStep
  dz [m/s] : Inport  Port=6  SampleTime=TimeStep
  R [rad] : Inport  Port=7  SampleTime=TimeStep
  P [rad] : Inport  Port=8  SampleTime=TimeStep
  Y [rad] : Inport  Port=9  SampleTime=TimeStep
  Constant : Constant  DisableCoverage=on  Value=positioningmode
  Discrete-Time Integrator : DiscreteIntegrator  SampleTime=TimeStep  ICPrevOutput=DiscIntNeverNeededParam  ICPrevScaledInput=DiscIntNeverNeededParam
  Ground : Ground
  Ground1 : Ground
  Mux1 : Mux  Inputs=[3 3]
  Mux2 : Mux  Inputs=3
  Mux3 : Mux  Inputs=3
  Mux4 : Mux  Inputs=3
  Mux5 : Mux  Inputs=[3 3]
  Mux6 : Mux  Inputs=[6 3]
  Switch : Switch  Threshold=0.5  SaturateOnIntegerOverflow=off  InputSameDT=off
  Transformation_BODY2GLOBAL : PreScanSimulinkLibrary/Simple_Vehicle_Dynamics/Chassis/MuxDynState/Transformation_BODY2GLOBAL  SystemSampleTime=-1  VariantActivationTime=update diagram  Latency=0  AutoFrameSizeCalculation=off
  mux3 : Mux  Inputs=3
  state : Outport
  wires:
  Constant/1 -> Switch/2
  Mux6/1 -> state/1
  Mux4/1 -> Mux1/1
  Mux5/1 -> Switch/3
  Mux1/1 -> Switch/1
  Switch/1 -> Mux6/1  "PosVeh wrt  GLOB"
  P [rad]/1 -> Mux3/2
  R [rad]/1 -> Mux3/1
  dz [m/s]/1 -> Mux2/3
  dy [m/s]/1 -> Mux2/2
  dx [m/s]/1 -> Mux2/1
  z [m]/1 -> Mux4/3
  y [m]/1 -> Mux4/2
  x [m]/1 -> Mux4/1
  Ground1/1 -> mux3/2  "pitch"
  Y [rad]/1 -> mux3/3, Mux3/3  "yaw"
  Mux3/1 -> Mux6/2
  Transformation_BODY2GLOBAL/1 -> Discrete-Time Integrator/1, Mux5/2  "VelVEH wrt  GLOB"
  mux3/1 -> Transformation_BODY2GLOBAL/2
  Ground/1 -> mux3/1  "roll"
  Mux2/1 -> Mux1/2, Transformation_BODY2GLOBAL/1
  Discrete-Time Integrator/1 -> Mux5/1  "PosVEH wrt  GLOB"

== system testemplanner_cs/Box_4/SELF_Demux/compas converter ==
  rotz [rad] : Inport
  cart2compas : Subsystem
  rad2deg : Gain  Gain=180/pi
  heading [deg] : Outport
  wires:
  rad2deg/1 -> cart2compas/1(Angle [deg])
  rotz [rad]/1 -> rad2deg/1
  cart2compas/1(heading [deg]) -> heading [deg]/1

== system testemplanner_cs/Box_5/Dynamics_Empty/MuxState ==
  note: mode: Dynamics
  note: mode: Positioning
  note: mode: Dynamics
      | VelVEHICLE
      | wrt VEH
  note: AnglesVEHICLE
      | wrtGLOB
  note: For state mode 'Dynamic' positions
      | are not taken into account, as they
      | are computed by integrating velocity.
      | Click annotation for Help.
  x [m] : Inport  SampleTime=TimeStep
  y [m] : Inport  Port=2  SampleTime=TimeStep
  z [m] : Inport  Port=3  SampleTime=TimeStep
  dx [m/s] : Inport  Port=4  SampleTime=TimeStep
  dy [m/s] : Inport  Port=5  SampleTime=TimeStep
  dz [m/s] : Inport  Port=6  SampleTime=TimeStep
  R [rad] : Inport  Port=7  SampleTime=TimeStep
  P [rad] : Inport  Port=8  SampleTime=TimeStep
  Y [rad] : Inport  Port=9  SampleTime=TimeStep
  Constant : Constant  DisableCoverage=on  Value=positioningmode
  Discrete-Time Integrator : DiscreteIntegrator  SampleTime=TimeStep  ICPrevOutput=DiscIntNeverNeededParam  ICPrevScaledInput=DiscIntNeverNeededParam
  Ground : Ground
  Ground1 : Ground
  Mux1 : Mux  Inputs=[3 3]
  Mux2 : Mux  Inputs=3
  Mux3 : Mux  Inputs=3
  Mux4 : Mux  Inputs=3
  Mux5 : Mux  Inputs=[3 3]
  Mux6 : Mux  Inputs=[6 3]
  Switch : Switch  Threshold=0.5  SaturateOnIntegerOverflow=off  InputSameDT=off
  Transformation_BODY2GLOBAL : PreScanSimulinkLibrary/Simple_Vehicle_Dynamics/Chassis/MuxDynState/Transformation_BODY2GLOBAL  SystemSampleTime=-1  VariantActivationTime=update diagram  Latency=0  AutoFrameSizeCalculation=off
  mux3 : Mux  Inputs=3
  state : Outport
  wires:
  Constant/1 -> Switch/2
  Mux6/1 -> state/1
  Mux4/1 -> Mux1/1
  Mux5/1 -> Switch/3
  Mux1/1 -> Switch/1
  Switch/1 -> Mux6/1  "PosVeh wrt  GLOB"
  P [rad]/1 -> Mux3/2
  R [rad]/1 -> Mux3/1
  dz [m/s]/1 -> Mux2/3
  dy [m/s]/1 -> Mux2/2
  dx [m/s]/1 -> Mux2/1
  z [m]/1 -> Mux4/3
  y [m]/1 -> Mux4/2
  x [m]/1 -> Mux4/1
  Ground1/1 -> mux3/2  "pitch"
  Y [rad]/1 -> mux3/3, Mux3/3  "yaw"
  Mux3/1 -> Mux6/2
  Transformation_BODY2GLOBAL/1 -> Discrete-Time Integrator/1, Mux5/2  "VelVEH wrt  GLOB"
  mux3/1 -> Transformation_BODY2GLOBAL/2
  Ground/1 -> mux3/1  "roll"
  Mux2/1 -> Mux1/2, Transformation_BODY2GLOBAL/1
  Discrete-Time Integrator/1 -> Mux5/1  "PosVEH wrt  GLOB"

== system testemplanner_cs/Box_5/SELF_Demux/compas converter ==
  rotz [rad] : Inport
  cart2compas : Subsystem
  rad2deg : Gain  Gain=180/pi
  heading [deg] : Outport
  wires:
  rad2deg/1 -> cart2compas/1(Angle [deg])
  rotz [rad]/1 -> rad2deg/1
  cart2compas/1(heading [deg]) -> heading [deg]/1

== system testemplanner_cs/Box_6/Dynamics_Empty/MuxState ==
  note: mode: Dynamics
  note: mode: Positioning
  note: mode: Dynamics
      | VelVEHICLE
      | wrt VEH
  note: AnglesVEHICLE
      | wrtGLOB
  note: For state mode 'Dynamic' positions
      | are not taken into account, as they
      | are computed by integrating velocity.
      | Click annotation for Help.
  x [m] : Inport  SampleTime=TimeStep
  y [m] : Inport  Port=2  SampleTime=TimeStep
  z [m] : Inport  Port=3  SampleTime=TimeStep
  dx [m/s] : Inport  Port=4  SampleTime=TimeStep
  dy [m/s] : Inport  Port=5  SampleTime=TimeStep
  dz [m/s] : Inport  Port=6  SampleTime=TimeStep
  R [rad] : Inport  Port=7  SampleTime=TimeStep
  P [rad] : Inport  Port=8  SampleTime=TimeStep
  Y [rad] : Inport  Port=9  SampleTime=TimeStep
  Constant : Constant  DisableCoverage=on  Value=positioningmode
  Discrete-Time Integrator : DiscreteIntegrator  SampleTime=TimeStep  ICPrevOutput=DiscIntNeverNeededParam  ICPrevScaledInput=DiscIntNeverNeededParam
  Ground : Ground
  Ground1 : Ground
  Mux1 : Mux  Inputs=[3 3]
  Mux2 : Mux  Inputs=3
  Mux3 : Mux  Inputs=3
  Mux4 : Mux  Inputs=3
  Mux5 : Mux  Inputs=[3 3]
  Mux6 : Mux  Inputs=[6 3]
  Switch : Switch  Threshold=0.5  SaturateOnIntegerOverflow=off  InputSameDT=off
  Transformation_BODY2GLOBAL : PreScanSimulinkLibrary/Simple_Vehicle_Dynamics/Chassis/MuxDynState/Transformation_BODY2GLOBAL  SystemSampleTime=-1  VariantActivationTime=update diagram  Latency=0  AutoFrameSizeCalculation=off
  mux3 : Mux  Inputs=3
  state : Outport
  wires:
  Constant/1 -> Switch/2
  Mux6/1 -> state/1
  Mux4/1 -> Mux1/1
  Mux5/1 -> Switch/3
  Mux1/1 -> Switch/1
  Switch/1 -> Mux6/1  "PosVeh wrt  GLOB"
  P [rad]/1 -> Mux3/2
  R [rad]/1 -> Mux3/1
  dz [m/s]/1 -> Mux2/3
  dy [m/s]/1 -> Mux2/2
  dx [m/s]/1 -> Mux2/1
  z [m]/1 -> Mux4/3
  y [m]/1 -> Mux4/2
  x [m]/1 -> Mux4/1
  Ground1/1 -> mux3/2  "pitch"
  Y [rad]/1 -> mux3/3, Mux3/3  "yaw"
  Mux3/1 -> Mux6/2
  Transformation_BODY2GLOBAL/1 -> Discrete-Time Integrator/1, Mux5/2  "VelVEH wrt  GLOB"
  mux3/1 -> Transformation_BODY2GLOBAL/2
  Ground/1 -> mux3/1  "roll"
  Mux2/1 -> Mux1/2, Transformation_BODY2GLOBAL/1
  Discrete-Time Integrator/1 -> Mux5/1  "PosVEH wrt  GLOB"

== system testemplanner_cs/Box_6/SELF_Demux/compas converter ==
  rotz [rad] : Inport
  cart2compas : Subsystem
  rad2deg : Gain  Gain=180/pi
  heading [deg] : Outport
  wires:
  rad2deg/1 -> cart2compas/1(Angle [deg])
  rotz [rad]/1 -> rad2deg/1
  cart2compas/1(heading [deg]) -> heading [deg]/1

== system testemplanner_cs/Audi_A8_Sedan_1/Dynamics_UserSpecified/CarSim2PreScanSTATE/Transformation_SprungMassCarSim2PreScan ==
  In1 : Inport
  Demux : Demux  Outputs=3
  Ini z-position VEHICLE wrt GLOBAL axis system [m] : Constant  Value=z0
  Mux : Mux  Inputs=3
  Sum1 : Sum  Inputs=+-
  Out1 : Outport
  wires:
  Mux/1 -> Out1/1
  Ini z-position VEHICLE wrt GLOBAL axis system [m]/1 -> Sum1/2
  Demux/1 -> Mux/1
  Sum1/1 -> Mux/3
  Demux/3 -> Sum1/1
  Demux/2 -> Mux/2
  In1/1 -> Demux/1

== system testemplanner_cs/Audi_A8_Sedan_1/SELF_Demux/compas converter/cart2compas ==
  Angle [deg] : Inport
  Constant : Constant  Value=90
  Constant1 : Constant  Value=360
  Gain : Gain  Gain=1/360
  Gain1 : Gain  Gain=360
  Gain2 : Gain  Gain=-1
  Rounding Function : Rounding
  Sum : Sum  Inputs=|-+
  Sum1 : Sum  Inputs=-+|
  Sum2 : Sum  Inputs=++|
  heading [deg] : Outport
  wires:
  Gain/1 -> Rounding Function/1
  Rounding Function/1 -> Gain1/1
  Gain1/1 -> Sum/1
  Angle [deg]/1 -> Sum1/2
  Sum/1 -> Gain2/1
  Sum1/1 -> Gain/1, Sum/2
  Constant/1 -> Sum1/1
  Gain2/1 -> Sum2/2
  Constant1/1 -> Sum2/1
  Sum2/1 -> heading [deg]/1

== system testemplanner_cs/Audi_A8_Sedan_1/control module/control main/chassic steering system ==
  LQR_final_angle : Inport
  Constant : Constant  Value=la
  Constant1 : Constant  Value=lb
  Constant17 : Constant  Value=c_factor
  Divide : Product  Inputs=*/
  Gain3 : Gain  Gain=180/pi
  Gain4 : Gain  Gain=360
  MATLAB Function : MATLAB Function  TreatAsAtomicUnit=on
  Saturation : Saturate  UpperLimit=70  LowerLimit=-70
  Saturation1 : Saturate  UpperLimit=1.2217  LowerLimit=-1.2217
  transfer wheel angle to rack displancement : Lookup_n-D  NumberOfTableDimensions=1  BreakpointsForDimension1=right_wheel_ground  Table=rack_displacement  InternalRulePriority=Speed  RndMeth=Simplest
  lat_steer_sw[deg] : Outport
  wires:
  Gain3/1 -> Saturation/1
  transfer wheel angle to rack displancement/1 -> Divide/1
  Constant17/1 -> Divide/2
  Gain4/1 -> lat_steer_sw[deg]/1
  Divide/1 -> Gain4/1
  Saturation/1 -> transfer wheel angle to rack displancement/1
  MATLAB Function/1(right_steer) -> Gain3/1
  Saturation1/1 -> MATLAB Function/1(u)
  LQR_final_angle/1 -> Saturation1/1
  Constant1/1 -> MATLAB Function/3(lb)
  Constant/1 -> MATLAB Function/2(la)
